simulink model "simulator"  (R2024a)
settings: Solver=VariableStepAuto  StartTime=0.0  StopTime=10  RelTol=1e-3
undefined symbols (not defined in the file): desiredState, gains, params, x0
libraries: simulink x2, matrix_library x1
settings Model: Creator=matteocolussi  LastModifiedBy=matteocolussi

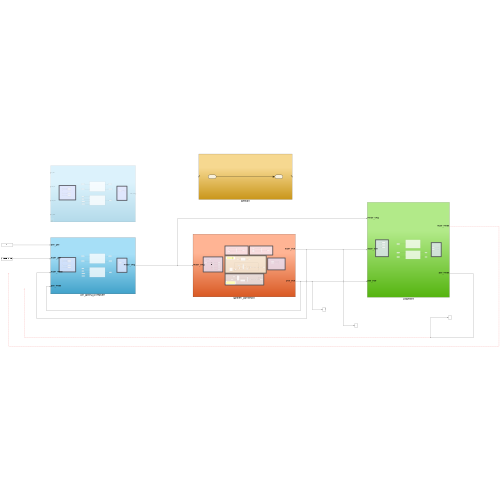
[thumbnail: Simulink's stored preview of the top-level diagram]
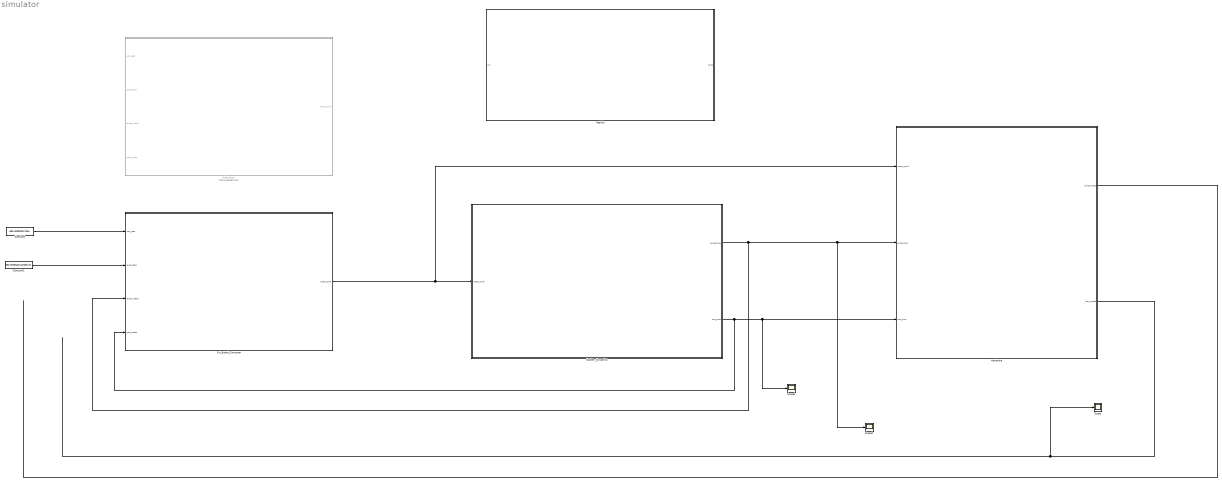
== system simulator ==
  Constant : Constant  Value=desiredState.rDes
  Constant1 : Constant  Value=desiredState.attDes(3)
  Hardware : Subsystem
  On_Board_Computer : Subsystem
  Results : Subsystem
  Scope : Scope
  Scope1 : Scope
  Scope2 : Scope
  Subsystem : Subsystem  Commented=on
  System_Dynamics : Subsystem
  wires:
  System_Dynamics/1(euler_true) -> On_Board_Computer/3(euler_meas), Hardware/2(euler_true), Scope2/1
  System_Dynamics/2(pos_true) -> On_Board_Computer/4(pos_meas), Hardware/3(pos_true), Scope1/1
  Hardware/1(euler_meas) -> ?
  Hardware/2(pos_meas) -> Scope/1
  Constant/1 -> On_Board_Computer/1(pos_des)
  Constant1/1 -> On_Board_Computer/2(euler_des)
  On_Board_Computer/1(motor_cmd) -> System_Dynamics/1(motor_cmd), Hardware/1(motor_cmd)

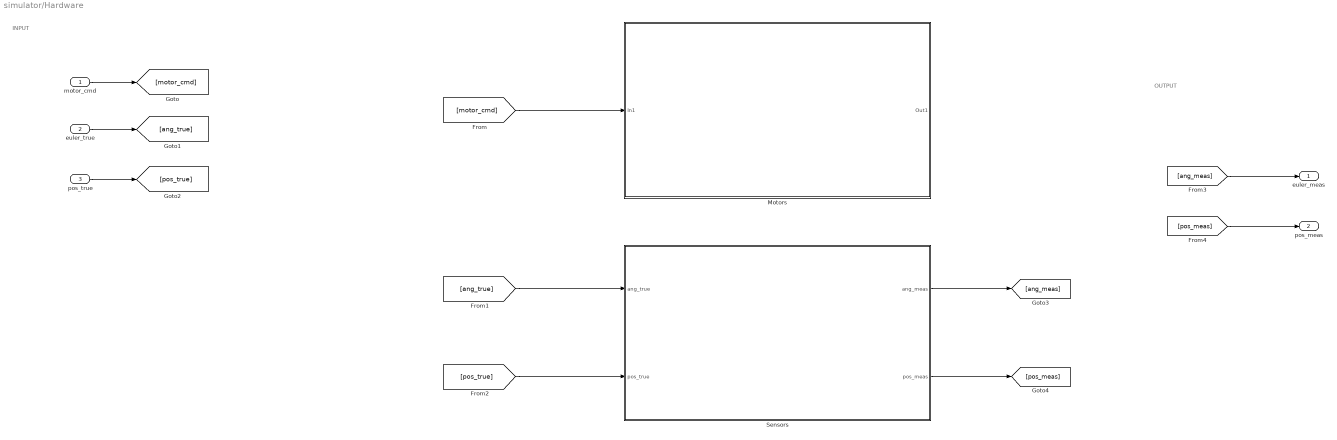
== system simulator/Hardware ==
  note: INPUT
  note: OUTPUT
  motor_cmd : Inport
  euler_true : Inport  Port=2
  pos_true : Inport  Port=3
  Motors : Subsystem
  Sensors : Subsystem
  euler_meas : Outport
  pos_meas : Outport  Port=2
  wires:
  motor_cmd/1 -> [motor_cmd]
  [motor_cmd] -> Motors/1(In1)
  euler_true/1 -> [ang_true]
  pos_true/1 -> [pos_true]
  [ang_true] -> Sensors/1(ang_true)
  [pos_true] -> Sensors/2(pos_true)
  Sensors/1(ang_meas) -> [ang_meas]
  Sensors/2(pos_meas) -> [pos_meas]
  [ang_meas] -> euler_meas/1
  [pos_meas] -> pos_meas/1

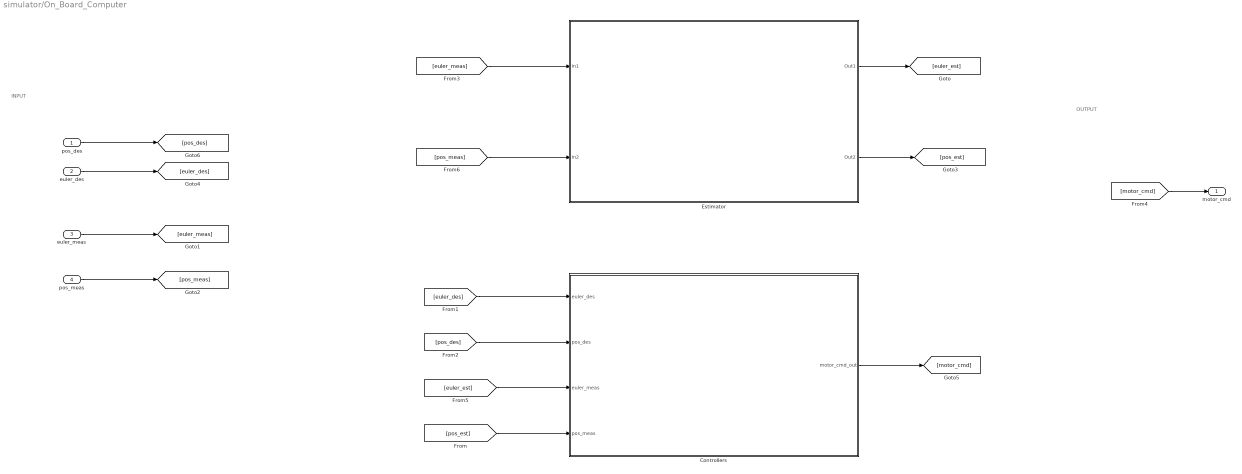
== system simulator/On_Board_Computer ==
  note: INPUT
  note: OUTPUT
  pos_des : Inport
  euler_des : Inport  Port=2
  euler_meas : Inport  Port=3
  pos_meas : Inport  Port=4
  Controllers : Subsystem
  Estimator : Subsystem
  motor_cmd : Outport
  wires:
  [euler_des] -> Controllers/1(euler_des)
  pos_des/1 -> [pos_des]
  pos_meas/1 -> [pos_meas]
  [pos_meas] -> Estimator/2(In2)
  [euler_meas] -> Estimator/1(In1)
  [pos_est] -> Controllers/4(pos_meas)
  euler_meas/1 -> [euler_meas]
  [motor_cmd] -> motor_cmd/1
  euler_des/1 -> [euler_des]
  [pos_des] -> Controllers/2(pos_des)
  Estimator/2(Out2) -> [pos_est]
  Estimator/1(Out1) -> [euler_est]
  [euler_est] -> Controllers/3(euler_meas)
  Controllers/1(motor_cmd_out) -> [motor_cmd]

== system simulator/Results ==
  In1 : Inport
  Out1 : Outport
  wires:
  In1/1 -> Out1/1

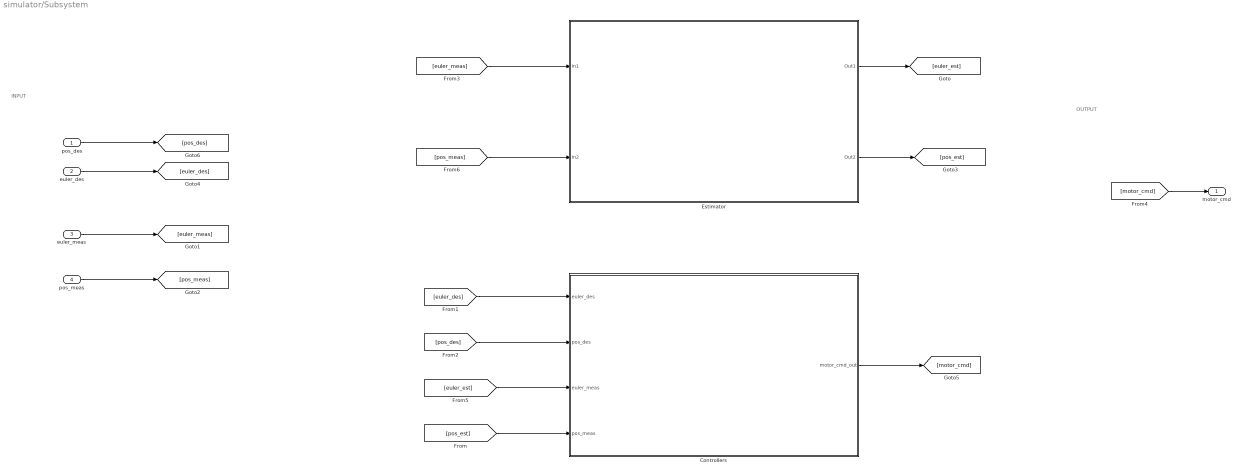
== system simulator/Subsystem ==
  note: INPUT
  note: OUTPUT
  pos_des : Inport
  euler_des : Inport  Port=2
  euler_meas : Inport  Port=3
  pos_meas : Inport  Port=4
  Controllers : Subsystem
  Estimator : Subsystem
  motor_cmd : Outport
  wires:
  [euler_des] -> Controllers/1(euler_des)
  pos_des/1 -> [pos_des]
  pos_meas/1 -> [pos_meas]
  [pos_meas] -> Estimator/2(In2)
  [euler_meas] -> Estimator/1(In1)
  [pos_est] -> Controllers/4(pos_meas)
  euler_meas/1 -> [euler_meas]
  [motor_cmd] -> motor_cmd/1
  euler_des/1 -> [euler_des]
  [pos_des] -> Controllers/2(pos_des)
  Estimator/2(Out2) -> [pos_est]
  Estimator/1(Out1) -> [euler_est]
  [euler_est] -> Controllers/3(euler_meas)
  Controllers/1(motor_cmd_out) -> [motor_cmd]

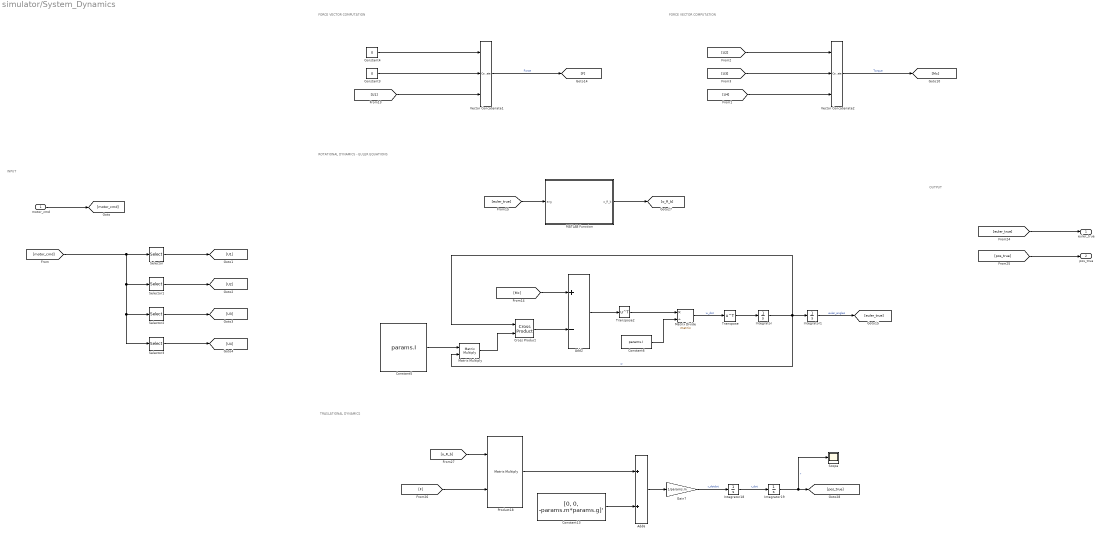
== system simulator/System_Dynamics ==
  note: ROTATIONAL DYNAMICS - EULER EQUATIONS
  note: FORCE VECTOR COMPUTATION
  note: INPUT
  note: OUTPUT
  note: TRASLATIONAL DYNAMICS
  note: FORCE VECTOR COMPUTATION
  motor_cmd : Inport
  Add2 : Sum  Inputs=+-
  Add6 : Sum
  Constant13 : Constant  Value=[0, 0, -params.m*params.g]'
  Constant3 : Constant  Value=0
  Constant4 : Constant  Value=0
  Constant5 : Constant  Value=params.I  VectorParams1D=off
  Constant6 : Constant  Value=params.I
  Cross Product : matrix_library/Cross Product
  Gain7 : Gain  Gain=1/params.m
  Integrator : Integrator
  Integrator1 : Integrator  InitialCondition=x0(7:9)
  Integrator18 : Integrator
  Integrator19 : Integrator  InitialCondition=x0(1:3);
  MATLAB Function : MATLAB Function  TreatAsAtomicUnit=on
  Matrix Divide : Product  Inputs=*/  Multiplication=Matrix(*)
  Matrix Multiply : Product  Multiplication=Matrix(*)
  Product18 : Product  Multiplication=Matrix(*)
  Scope : Scope
  Selector : Selector  InputPortWidth=4  IndexOptions=Index vector (dialog)  Indices=1  OutputSizes=1
  Selector1 : Selector  InputPortWidth=4  IndexOptions=Index vector (dialog)  Indices=2  OutputSizes=1
  Selector2 : Selector  InputPortWidth=4  IndexOptions=Index vector (dialog)  Indices=3  OutputSizes=1
  Selector3 : Selector  InputPortWidth=4  IndexOptions=Index vector (dialog)  Indices=4  OutputSizes=1
  Transpose : Math  Operator=transpose
  Transpose2 : Math  Operator=transpose
  Vector Concatenate1 : Concatenate  NumInputs=3
  Vector Concatenate2 : Concatenate  NumInputs=3
  euler_true : Outport
  pos_true : Outport  Port=2
  wires:
  motor_cmd/1 -> [motor_cmd]
  Selector/1 -> [U1]
  Selector1/1 -> [U2]
  Selector2/1 -> [U3]
  [motor_cmd] -> Selector3/1, Selector2/1, Selector1/1, Selector/1
  Selector3/1 -> [U4]
  [U1] -> Vector Concatenate1/3
  Constant3/1 -> Vector Concatenate1/2
  Constant4/1 -> Vector Concatenate1/1
  Vector Concatenate1/1 -> [F]  "Force"
  [euler_true] -> MATLAB Function/1(ang)
  MATLAB Function/1(o_R_b) -> [o_R_b]
  [euler_true] -> euler_true/1
  [pos_true] -> pos_true/1
  Add6/1 -> Gain7/1
  [F] -> Product18/2
  Product18/1 -> Add6/1
  Gain7/1 -> Integrator18/1  "r_dotdot"
  [o_R_b] -> Product18/1
  Constant13/1 -> Add6/2
  Integrator18/1 -> Integrator19/1  "r_dot"
  Integrator19/1 -> [pos_true], Scope/1  "r"
  Constant5/1 -> Matrix Multiply/1
  Matrix Multiply/1 -> Cross Product/2
  Cross Product/1 -> Add2/2
  Add2/1 -> Transpose2/1
  Constant6/1 -> Matrix Divide/2
  Matrix Divide/1 -> Transpose/1  "w_dot"
  Integrator/1 -> Integrator1/1, Cross Product/1, Matrix Multiply/2  "w"
  Integrator1/1 -> [euler_true]  "euler_angles"
  [U2] -> Vector Concatenate2/1
  Vector Concatenate2/1 -> [Mc]  "Torque"
  [U4] -> Vector Concatenate2/3
  [U3] -> Vector Concatenate2/2
  Transpose/1 -> Integrator/1
  [Mc] -> Add2/1
  Transpose2/1 -> Matrix Divide/1

== system simulator/Hardware/Motors ==
  In1 : Inport
  Out1 : Outport
  wires:
  In1/1 -> Out1/1

== system simulator/Hardware/Sensors ==
  note: OUTPUT
  note: INPUT
  ang_true : Inport
  pos_true : Inport  Port=2
  MPU6050 : Subsystem
  ang_meas : Outport
  pos_meas : Outport  Port=2
  wires:
  ang_true/1 -> [ang_true]
  pos_true/1 -> [pos_true]
  [ang_meas] -> ang_meas/1
  [pos_meas] -> pos_meas/1
  [ang_true] -> MPU6050/1(ang_true)
  [pos_true] -> MPU6050/2(pos_true)
  MPU6050/1(ang_meas) -> [ang_meas]
  MPU6050/2(pos_meas) -> [pos_meas]

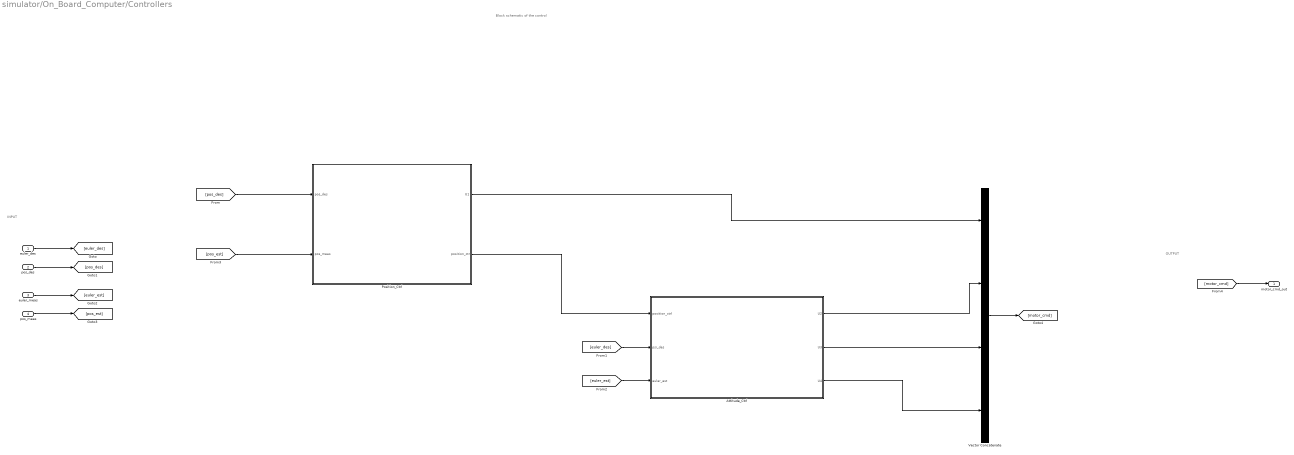
== system simulator/On_Board_Computer/Controllers ==
  note: Block schematic of the control
  note: OUTPUT
  note: INPUT
  euler_des : Inport
  pos_des : Inport  Port=2
  euler_meas : Inport  Port=3
  pos_meas : Inport  Port=4
  Attitude_Ctrl : Subsystem
  Position_Ctrl : Subsystem
  Vector Concatenate : Concatenate  NumInputs=4
  motor_cmd_out : Outport
  wires:
  euler_des/1 -> [euler_des]
  pos_des/1 -> [pos_des]
  pos_meas/1 -> [pos_est]
  euler_meas/1 -> [euler_est]
  [euler_est] -> Attitude_Ctrl/3(euler_est)
  [motor_cmd] -> motor_cmd_out/1
  [pos_est] -> Position_Ctrl/2(pos_meas)
  [pos_des] -> Position_Ctrl/1(pos_des)
  Position_Ctrl/2(position_ctrl) -> Attitude_Ctrl/1(position_ctrl)
  Position_Ctrl/1(U1) -> Vector Concatenate/1
  Attitude_Ctrl/1(U2) -> Vector Concatenate/2
  Attitude_Ctrl/2(U3) -> Vector Concatenate/3
  Attitude_Ctrl/3(U4) -> Vector Concatenate/4
  Vector Concatenate/1 -> [motor_cmd]
  [euler_des] -> Attitude_Ctrl/2(psi_des)

== system simulator/On_Board_Computer/Estimator ==
  In1 : Inport
  In2 : Inport  Port=2
  Out1 : Outport
  Out2 : Outport  Port=2
  wires:
  In1/1 -> Out1/1
  In2/1 -> Out2/1

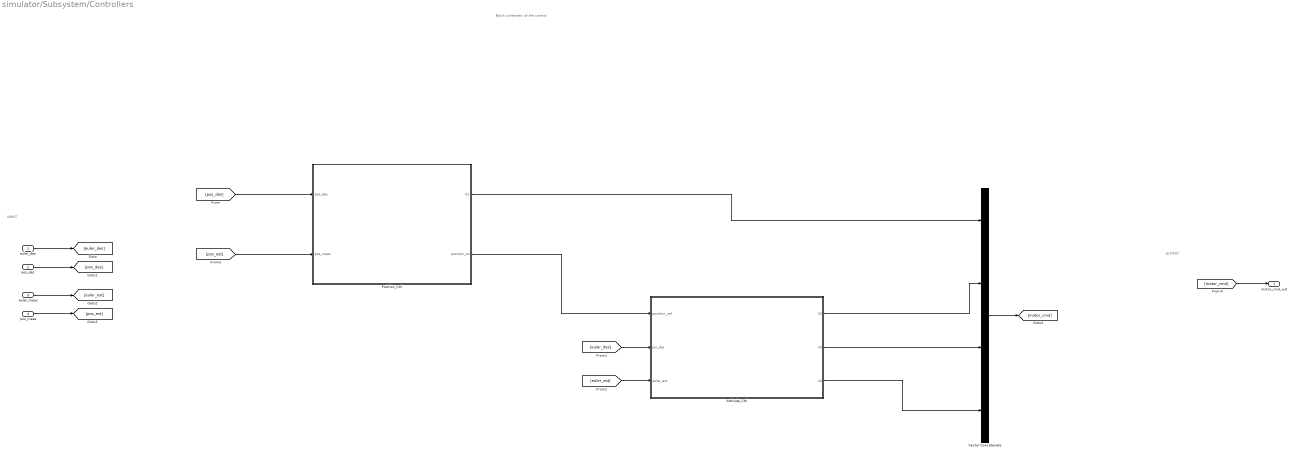
== system simulator/Subsystem/Controllers ==
  note: Block schematic of the control
  note: OUTPUT
  note: INPUT
  euler_des : Inport
  pos_des : Inport  Port=2
  euler_meas : Inport  Port=3
  pos_meas : Inport  Port=4
  Attitude_Ctrl : Subsystem
  Position_Ctrl : Subsystem
  Vector Concatenate : Concatenate  NumInputs=4
  motor_cmd_out : Outport
  wires:
  euler_des/1 -> [euler_des]
  pos_des/1 -> [pos_des]
  pos_meas/1 -> [pos_est]
  euler_meas/1 -> [euler_est]
  [euler_est] -> Attitude_Ctrl/3(euler_est)
  [motor_cmd] -> motor_cmd_out/1
  [pos_est] -> Position_Ctrl/2(pos_meas)
  [pos_des] -> Position_Ctrl/1(pos_des)
  Position_Ctrl/2(position_ctrl) -> Attitude_Ctrl/1(position_ctrl)
  Position_Ctrl/1(U1) -> Vector Concatenate/1
  Attitude_Ctrl/1(U2) -> Vector Concatenate/2
  Attitude_Ctrl/2(U3) -> Vector Concatenate/3
  Attitude_Ctrl/3(U4) -> Vector Concatenate/4
  Vector Concatenate/1 -> [motor_cmd]
  [euler_des] -> Attitude_Ctrl/2(psi_des)

== system simulator/Subsystem/Estimator ==
  In1 : Inport
  In2 : Inport  Port=2
  Out1 : Outport
  Out2 : Outport  Port=2
  wires:
  In1/1 -> Out1/1
  In2/1 -> Out2/1

== system simulator/Hardware/Sensors/MPU6050 ==
  note: INPUT
  note: OUTPUT
  ang_true : Inport
  pos_true : Inport  Port=2
  ACCELEROMETER : Subsystem
  GYROSCOPE : Subsystem
  ang_meas : Outport
  pos_meas : Outport  Port=2
  wires:
  ang_true/1 -> [ang_true]
  pos_true/1 -> [pos_true]
  [pos_meas] -> pos_meas/1
  [ang_meas] -> ang_meas/1
  [ang_true] -> GYROSCOPE/1(ang_true)
  [pos_true] -> ACCELEROMETER/1(pos_true)
  GYROSCOPE/1(ang_meas) -> [ang_meas]
  ACCELEROMETER/1(pos_meas) -> [pos_meas]

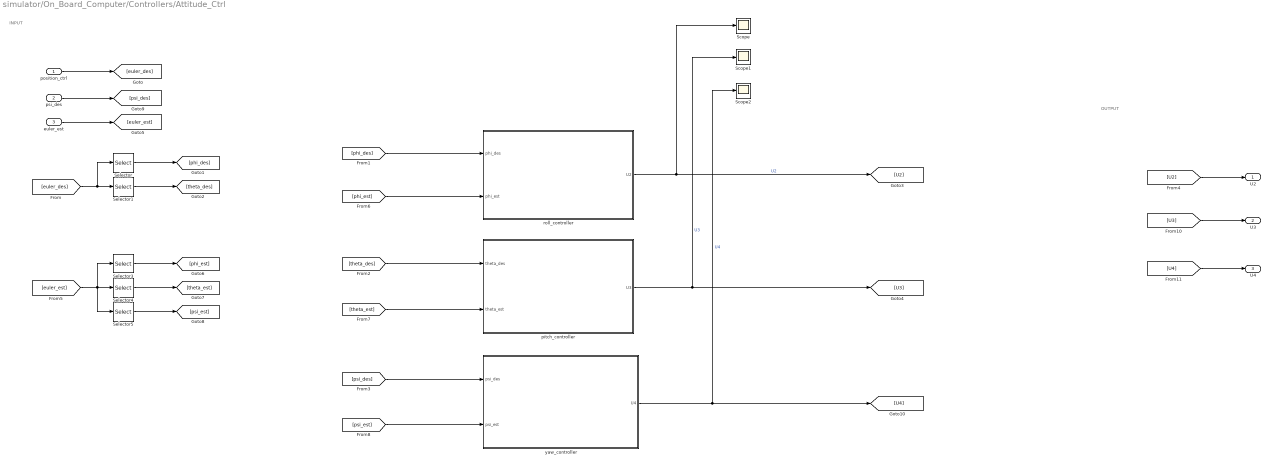
== system simulator/On_Board_Computer/Controllers/Attitude_Ctrl ==
  note: OUTPUT
  note: INPUT
  position_ctrl : Inport
  psi_des : Inport  Port=2
  euler_est : Inport  Port=3
  Scope : Scope
  Scope1 : Scope
  Scope2 : Scope
  Selector : Selector  InputPortWidth=2  IndexOptions=Index vector (dialog)  Indices=1  OutputSizes=1
  Selector1 : Selector  InputPortWidth=2  IndexOptions=Index vector (dialog)  Indices=2  OutputSizes=1
  Selector3 : Selector  InputPortWidth=3  IndexOptions=Index vector (dialog)  Indices=1  OutputSizes=1
  Selector4 : Selector  InputPortWidth=3  IndexOptions=Index vector (dialog)  Indices=2  OutputSizes=1
  Selector5 : Selector  InputPortWidth=3  IndexOptions=Index vector (dialog)  Indices=3  OutputSizes=1
  pitch_controller : Subsystem
  roll_controller : Subsystem
  yaw_controller : Subsystem
  U2 : Outport
  U3 : Outport  Port=2
  U4 : Outport  Port=3
  wires:
  position_ctrl/1 -> [euler_des]
  [phi_des] -> roll_controller/1(phi_des)
  [theta_des] -> pitch_controller/1(theta_des)
  [psi_des] -> yaw_controller/1(psi_des)
  roll_controller/1(U2) -> [U2], Scope/1  "U2"
  pitch_controller/1(U3) -> [U3], Scope1/1  "U3"
  yaw_controller/1(U4) -> [U4], Scope2/1  "U4"
  euler_est/1 -> [euler_est]
  [phi_est] -> roll_controller/2(phi_est)
  [theta_est] -> pitch_controller/2(theta_est)
  [psi_est] -> yaw_controller/2(psi_est)
  Selector/1 -> [phi_des]
  [euler_des] -> Selector1/1, Selector/1
  Selector1/1 -> [theta_des]
  [euler_est] -> Selector5/1, Selector4/1, Selector3/1
  Selector4/1 -> [theta_est]
  Selector5/1 -> [psi_est]
  Selector3/1 -> [phi_est]
  [U2] -> U2/1
  [U3] -> U3/1
  [U4] -> U4/1
  psi_des/1 -> [psi_des]

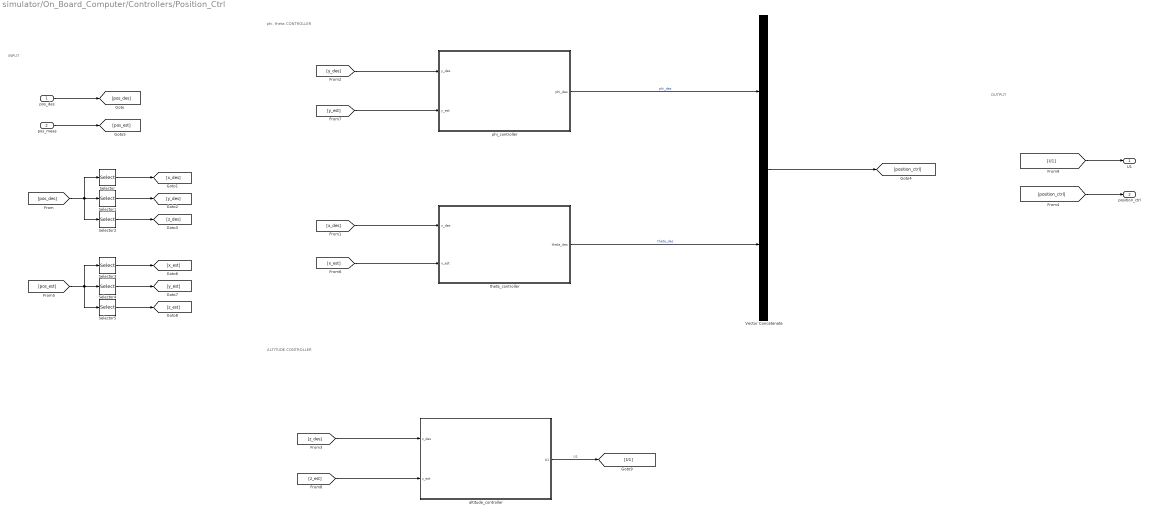
== system simulator/On_Board_Computer/Controllers/Position_Ctrl ==
  note: ALTITUDE CONTROLLER
  note: phi, theta CONTROLLER
  note: INPUT
  note: OUTPUT
  pos_des : Inport
  pos_meas : Inport  Port=2
  Selector : Selector  InputPortWidth=3  IndexOptions=Index vector (dialog)  Indices=1  OutputSizes=1
  Selector1 : Selector  InputPortWidth=3  IndexOptions=Index vector (dialog)  Indices=2  OutputSizes=1
  Selector2 : Selector  InputPortWidth=3  IndexOptions=Index vector (dialog)  Indices=3  OutputSizes=1
  Selector3 : Selector  InputPortWidth=3  IndexOptions=Index vector (dialog)  Indices=1  OutputSizes=1
  Selector4 : Selector  InputPortWidth=3  IndexOptions=Index vector (dialog)  Indices=2  OutputSizes=1
  Selector5 : Selector  InputPortWidth=3  IndexOptions=Index vector (dialog)  Indices=3  OutputSizes=1
  Vector Concatenate : Concatenate
  altitude_controller : Subsystem
  phi_controller : Subsystem
  theta_controller : Subsystem
  U1 : Outport
  position_ctrl : Outport  Port=2
  wires:
  Selector3/1 -> [x_est]
  Selector4/1 -> [y_est]
  [pos_est] -> Selector5/1, Selector4/1, Selector3/1
  pos_meas/1 -> [pos_est]
  Selector5/1 -> [z_est]
  [pos_des] -> Selector2/1, Selector1/1, Selector/1
  Selector/1 -> [x_des]
  pos_des/1 -> [pos_des]
  Selector1/1 -> [y_des]
  Selector2/1 -> [z_des]
  [y_est] -> phi_controller/2(y_est)
  [x_des] -> theta_controller/1(x_des)
  [y_des] -> phi_controller/1(y_des)
  [x_est] -> theta_controller/2(x_est)
  [position_ctrl] -> position_ctrl/1
  Vector Concatenate/1 -> [position_ctrl]
  theta_controller/1(theta_des) -> Vector Concatenate/2  "theta_des"
  [z_est] -> altitude_controller/2(z_est)
  [z_des] -> altitude_controller/1(z_des)
  altitude_controller/1(U1) -> [U1]  "U1"
  [U1] -> U1/1
  phi_controller/1(phi_des) -> Vector Concatenate/1  "phi_des"

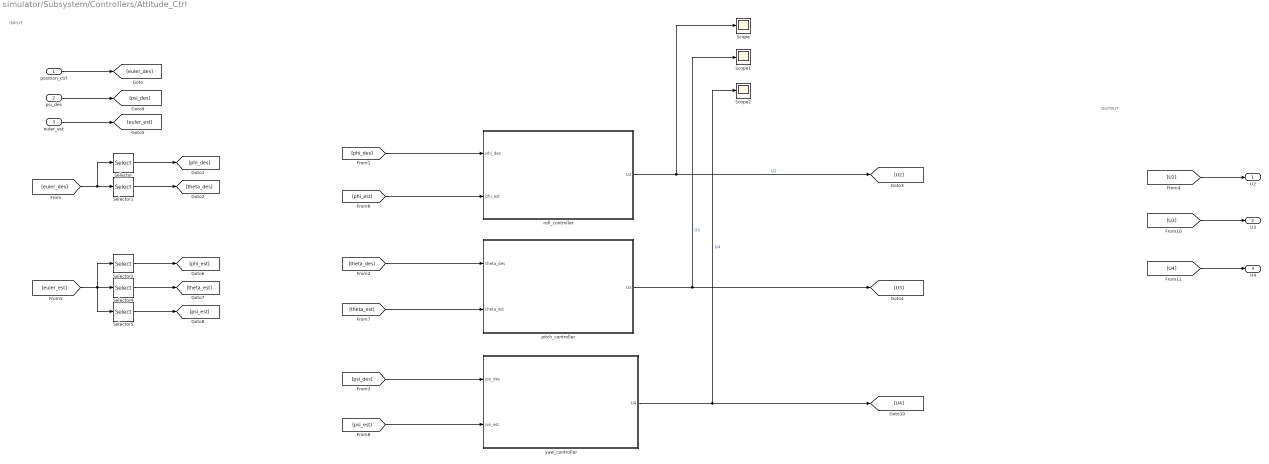
== system simulator/Subsystem/Controllers/Attitude_Ctrl ==
  note: OUTPUT
  note: INPUT
  position_ctrl : Inport
  psi_des : Inport  Port=2
  euler_est : Inport  Port=3
  Scope : Scope
  Scope1 : Scope
  Scope2 : Scope
  Selector : Selector  InputPortWidth=2  IndexOptions=Index vector (dialog)  Indices=1  OutputSizes=1
  Selector1 : Selector  InputPortWidth=2  IndexOptions=Index vector (dialog)  Indices=2  OutputSizes=1
  Selector3 : Selector  InputPortWidth=3  IndexOptions=Index vector (dialog)  Indices=1  OutputSizes=1
  Selector4 : Selector  InputPortWidth=3  IndexOptions=Index vector (dialog)  Indices=2  OutputSizes=1
  Selector5 : Selector  InputPortWidth=3  IndexOptions=Index vector (dialog)  Indices=3  OutputSizes=1
  pitch_controller : Subsystem
  roll_controller : Subsystem
  yaw_controller : Subsystem
  U2 : Outport
  U3 : Outport  Port=2
  U4 : Outport  Port=3
  wires:
  position_ctrl/1 -> [euler_des]
  [phi_des] -> roll_controller/1(phi_des)
  [theta_des] -> pitch_controller/1(theta_des)
  [psi_des] -> yaw_controller/1(psi_des)
  roll_controller/1(U2) -> [U2], Scope/1  "U2"
  pitch_controller/1(U3) -> [U3], Scope1/1  "U3"
  yaw_controller/1(U4) -> [U4], Scope2/1  "U4"
  euler_est/1 -> [euler_est]
  [phi_est] -> roll_controller/2(phi_est)
  [theta_est] -> pitch_controller/2(theta_est)
  [psi_est] -> yaw_controller/2(psi_est)
  Selector/1 -> [phi_des]
  [euler_des] -> Selector1/1, Selector/1
  Selector1/1 -> [theta_des]
  [euler_est] -> Selector5/1, Selector4/1, Selector3/1
  Selector4/1 -> [theta_est]
  Selector5/1 -> [psi_est]
  Selector3/1 -> [phi_est]
  [U2] -> U2/1
  [U3] -> U3/1
  [U4] -> U4/1
  psi_des/1 -> [psi_des]

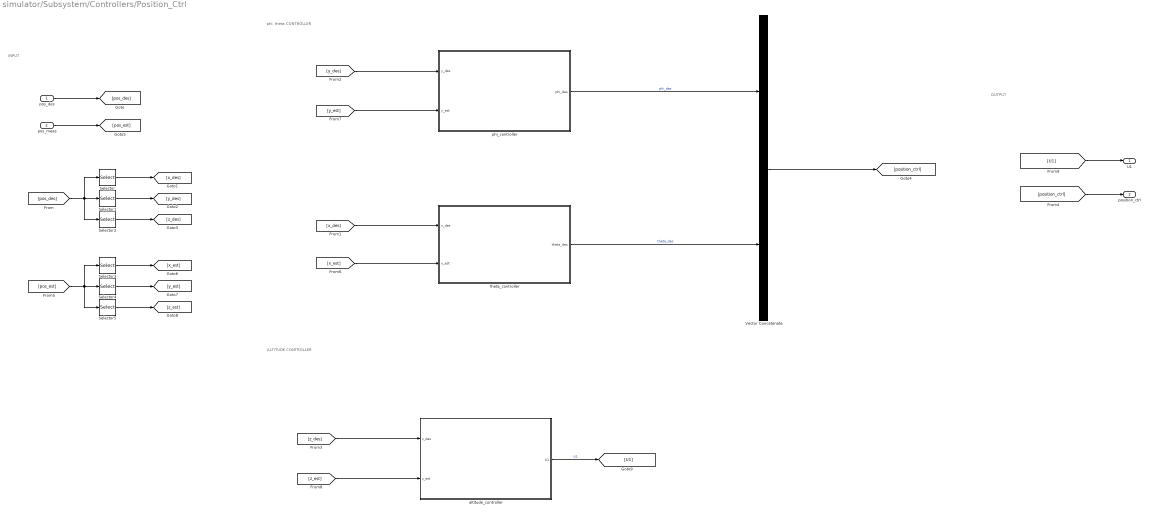
== system simulator/Subsystem/Controllers/Position_Ctrl ==
  note: ALTITUDE CONTROLLER
  note: phi, theta CONTROLLER
  note: INPUT
  note: OUTPUT
  pos_des : Inport
  pos_meas : Inport  Port=2
  Selector : Selector  InputPortWidth=3  IndexOptions=Index vector (dialog)  Indices=1  OutputSizes=1
  Selector1 : Selector  InputPortWidth=3  IndexOptions=Index vector (dialog)  Indices=2  OutputSizes=1
  Selector2 : Selector  InputPortWidth=3  IndexOptions=Index vector (dialog)  Indices=3  OutputSizes=1
  Selector3 : Selector  InputPortWidth=3  IndexOptions=Index vector (dialog)  Indices=1  OutputSizes=1
  Selector4 : Selector  InputPortWidth=3  IndexOptions=Index vector (dialog)  Indices=2  OutputSizes=1
  Selector5 : Selector  InputPortWidth=3  IndexOptions=Index vector (dialog)  Indices=3  OutputSizes=1
  Vector Concatenate : Concatenate
  altitude_controller : Subsystem
  phi_controller : Subsystem
  theta_controller : Subsystem
  U1 : Outport
  position_ctrl : Outport  Port=2
  wires:
  Selector3/1 -> [x_est]
  Selector4/1 -> [y_est]
  [pos_est] -> Selector5/1, Selector4/1, Selector3/1
  pos_meas/1 -> [pos_est]
  Selector5/1 -> [z_est]
  [pos_des] -> Selector2/1, Selector1/1, Selector/1
  Selector/1 -> [x_des]
  pos_des/1 -> [pos_des]
  Selector1/1 -> [y_des]
  Selector2/1 -> [z_des]
  [y_est] -> phi_controller/2(y_est)
  [x_des] -> theta_controller/1(x_des)
  [y_des] -> phi_controller/1(y_des)
  [x_est] -> theta_controller/2(x_est)
  [position_ctrl] -> position_ctrl/1
  Vector Concatenate/1 -> [position_ctrl]
  theta_controller/1(theta_des) -> Vector Concatenate/2  "theta_des"
  [z_est] -> altitude_controller/2(z_est)
  [z_des] -> altitude_controller/1(z_des)
  altitude_controller/1(U1) -> [U1]  "U1"
  [U1] -> U1/1
  phi_controller/1(phi_des) -> Vector Concatenate/1  "phi_des"

== system simulator/Hardware/Sensors/MPU6050/ACCELEROMETER ==
  pos_true : Inport
  Band-Limited White Noise : simulink/Sources/Band-Limited White Noise  Cov=[0.1]  Ts=0.1  seed=[23341]
  Sum : Sum  Inputs=|++
  pos_meas : Outport
  wires:
  Band-Limited White Noise/1 -> Sum/2
  pos_true/1 -> Sum/1
  Sum/1 -> pos_meas/1

== system simulator/Hardware/Sensors/MPU6050/GYROSCOPE ==
  ang_true : Inport
  Band-Limited White Noise : simulink/Sources/Band-Limited White Noise  Cov=[0.1]  Ts=0.1  seed=[23341]
  Sum : Sum  Inputs=|++
  ang_meas : Outport
  wires:
  ang_true/1 -> Sum/1
  Band-Limited White Noise/1 -> Sum/2
  Sum/1 -> ang_meas/1

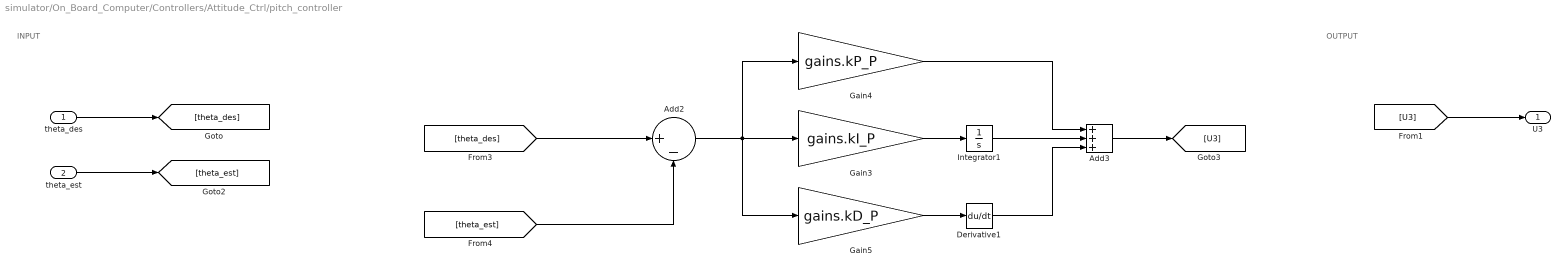
== system simulator/On_Board_Computer/Controllers/Attitude_Ctrl/pitch_controller ==
  note: OUTPUT
  note: INPUT
  theta_des : Inport
  theta_est : Inport  Port=2
  Add2 : Sum  Inputs=|+-
  Add3 : Sum  Inputs=+++
  Derivative1 : Derivative
  Gain3 : Gain  Gain=gains.kI_P
  Gain4 : Gain  Gain=gains.kP_P
  Gain5 : Gain  Gain=gains.kD_P
  Integrator1 : Integrator
  U3 : Outport
  wires:
  [U3] -> U3/1
  theta_des/1 -> [theta_des]
  theta_est/1 -> [theta_est]
  [theta_des] -> Add2/1
  Gain4/1 -> Add3/1
  Add3/1 -> [U3]
  Derivative1/1 -> Add3/3
  [theta_est] -> Add2/2
  Integrator1/1 -> Add3/2
  Add2/1 -> Gain5/1, Gain4/1, Gain3/1
  Gain5/1 -> Derivative1/1
  Gain3/1 -> Integrator1/1

== system simulator/On_Board_Computer/Controllers/Attitude_Ctrl/roll_controller ==
  note: OUTPUT
  note: INPUT
  phi_des : Inport
  phi_est : Inport  Port=2
  Add2 : Sum  Inputs=|+-
  Add3 : Sum  Inputs=+++
  Derivative1 : Derivative
  Gain3 : Gain  Gain=gains.kI_R
  Gain4 : Gain  Gain=gains.kP_R
  Gain5 : Gain  Gain=gains.kD_R
  Integrator1 : Integrator
  U2 : Outport
  wires:
  phi_des/1 -> [phi_des]
  [U2] -> U2/1
  phi_est/1 -> [phi_est]
  [phi_des] -> Add2/1
  Gain4/1 -> Add3/1
  Add3/1 -> [U2]
  Derivative1/1 -> Add3/3
  [phi_est] -> Add2/2
  Integrator1/1 -> Add3/2
  Add2/1 -> Gain5/1, Gain4/1, Gain3/1
  Gain5/1 -> Derivative1/1
  Gain3/1 -> Integrator1/1

== system simulator/On_Board_Computer/Controllers/Attitude_Ctrl/yaw_controller ==
  note: OUTPUT
  note: INPUT
  psi_des : Inport
  psi_est : Inport  Port=2
  Add2 : Sum  Inputs=|+-
  Add3 : Sum  Inputs=+++
  Derivative1 : Derivative
  Gain3 : Gain  Gain=gains.kI_Y
  Gain4 : Gain  Gain=gains.kP_Y
  Gain5 : Gain  Gain=gains.kD_Y
  Integrator1 : Integrator
  U4 : Outport
  wires:
  [U4] -> U4/1
  psi_des/1 -> [psi_des]
  psi_est/1 -> [psi_est]
  [psi_des] -> Add2/1
  Gain4/1 -> Add3/1
  Add3/1 -> [U4]
  Derivative1/1 -> Add3/3
  [psi_est] -> Add2/2
  Integrator1/1 -> Add3/2
  Add2/1 -> Gain5/1, Gain4/1, Gain3/1
  Gain5/1 -> Derivative1/1
  Gain3/1 -> Integrator1/1

== system simulator/On_Board_Computer/Controllers/Position_Ctrl/altitude_controller ==
  note: OUTPUT
  note: INPUT
  z_des : Inport
  z_est : Inport  Port=2
  Add2 : Sum  Inputs=|+-
  Add3 : Sum  Inputs=+++
  Derivative1 : Derivative
  Gain3 : Gain  Gain=gains.kI_T
  Gain4 : Gain  Gain=gains.kP_T
  Gain5 : Gain  Gain=gains.kD_T
  Integrator1 : Integrator
  U1 : Outport
  wires:
  [U1] -> U1/1
  z_des/1 -> [z_des]
  z_est/1 -> [z_est]
  [z_des] -> Add2/1
  Gain4/1 -> Add3/1
  Add3/1 -> [U1]
  Derivative1/1 -> Add3/3
  [z_est] -> Add2/2
  Integrator1/1 -> Add3/2
  Add2/1 -> Gain5/1, Gain4/1, Gain3/1
  Gain5/1 -> Derivative1/1
  Gain3/1 -> Integrator1/1

== system simulator/On_Board_Computer/Controllers/Position_Ctrl/phi_controller ==
  note: OUTPUT
  note: INPUT
  y_des : Inport
  y_est : Inport  Port=2
  Add : Sum  Inputs=|+-
  Add1 : Sum  Inputs=+++
  Derivative : Derivative
  Gain1 : Gain  Gain=gains.kI_phi
  Gain2 : Gain  Gain=gains.kP_phi
  Gain3 : Gain  Gain=gains.kD_phi
  Integrator : Integrator
  phi_des : Outport
  wires:
  [phi_des] -> phi_des/1
  [y_des] -> Add/1
  y_des/1 -> [y_des]
  y_est/1 -> [y_est]
  [y_est] -> Add/2
  Integrator/1 -> Add1/2
  Gain1/1 -> Integrator/1
  Add/1 -> Gain3/1, Gain2/1, Gain1/1
  Gain2/1 -> Add1/1
  Derivative/1 -> Add1/3
  Add1/1 -> [phi_des]
  Gain3/1 -> Derivative/1

== system simulator/On_Board_Computer/Controllers/Position_Ctrl/theta_controller ==
  note: OUTPUT
  note: INPUT
  x_des : Inport
  x_est : Inport  Port=2
  Add2 : Sum  Inputs=|+-
  Add3 : Sum  Inputs=+++
  Derivative1 : Derivative
  Gain3 : Gain  Gain=gains.kI_theta
  Gain4 : Gain  Gain=gains.kP_theta
  Gain5 : Gain  Gain=gains.kD_theta
  Integrator1 : Integrator
  theta_des : Outport
  wires:
  x_des/1 -> [x_des]
  [theta_des] -> theta_des/1
  x_est/1 -> [x_est]
  [x_des] -> Add2/1
  Gain4/1 -> Add3/1
  Add3/1 -> [theta_des]
  Derivative1/1 -> Add3/3
  [x_est] -> Add2/2
  Integrator1/1 -> Add3/2
  Add2/1 -> Gain5/1, Gain4/1, Gain3/1
  Gain5/1 -> Derivative1/1
  Gain3/1 -> Integrator1/1

== system simulator/Subsystem/Controllers/Attitude_Ctrl/pitch_controller ==
  note: OUTPUT
  note: INPUT
  theta_des : Inport
  theta_est : Inport  Port=2
  Add2 : Sum  Inputs=|+-
  Add3 : Sum  Inputs=+++
  Derivative1 : Derivative
  Gain3 : Gain  Gain=gains.kI_P
  Gain4 : Gain  Gain=gains.kP_P
  Gain5 : Gain  Gain=gains.kD_P
  Integrator1 : Integrator
  U3 : Outport
  wires:
  [U3] -> U3/1
  theta_des/1 -> [theta_des]
  theta_est/1 -> [theta_est]
  [theta_des] -> Add2/1
  Gain4/1 -> Add3/1
  Add3/1 -> [U3]
  Derivative1/1 -> Add3/3
  [theta_est] -> Add2/2
  Integrator1/1 -> Add3/2
  Add2/1 -> Gain5/1, Gain4/1, Gain3/1
  Gain5/1 -> Derivative1/1
  Gain3/1 -> Integrator1/1

== system simulator/Subsystem/Controllers/Attitude_Ctrl/roll_controller ==
  note: OUTPUT
  note: INPUT
  phi_des : Inport
  phi_est : Inport  Port=2
  Add2 : Sum  Inputs=|+-
  Add3 : Sum  Inputs=+++
  Derivative1 : Derivative
  Gain3 : Gain  Gain=gains.kI_R
  Gain4 : Gain  Gain=gains.kP_R
  Gain5 : Gain  Gain=gains.kD_R
  Integrator1 : Integrator
  U2 : Outport
  wires:
  phi_des/1 -> [phi_des]
  [U2] -> U2/1
  phi_est/1 -> [phi_est]
  [phi_des] -> Add2/1
  Gain4/1 -> Add3/1
  Add3/1 -> [U2]
  Derivative1/1 -> Add3/3
  [phi_est] -> Add2/2
  Integrator1/1 -> Add3/2
  Add2/1 -> Gain5/1, Gain4/1, Gain3/1
  Gain5/1 -> Derivative1/1
  Gain3/1 -> Integrator1/1

== system simulator/Subsystem/Controllers/Attitude_Ctrl/yaw_controller ==
  note: OUTPUT
  note: INPUT
  psi_des : Inport
  psi_est : Inport  Port=2
  Add2 : Sum  Inputs=|+-
  Add3 : Sum  Inputs=+++
  Derivative1 : Derivative
  Gain3 : Gain  Gain=gains.kI_Y
  Gain4 : Gain  Gain=gains.kP_Y
  Gain5 : Gain  Gain=gains.kD_Y
  Integrator1 : Integrator
  U4 : Outport
  wires:
  [U4] -> U4/1
  psi_des/1 -> [psi_des]
  psi_est/1 -> [psi_est]
  [psi_des] -> Add2/1
  Gain4/1 -> Add3/1
  Add3/1 -> [U4]
  Derivative1/1 -> Add3/3
  [psi_est] -> Add2/2
  Integrator1/1 -> Add3/2
  Add2/1 -> Gain5/1, Gain4/1, Gain3/1
  Gain5/1 -> Derivative1/1
  Gain3/1 -> Integrator1/1

== system simulator/Subsystem/Controllers/Position_Ctrl/altitude_controller ==
  note: OUTPUT
  note: INPUT
  z_des : Inport
  z_est : Inport  Port=2
  Add2 : Sum  Inputs=|+-
  Add3 : Sum  Inputs=+++
  Derivative1 : Derivative
  Gain3 : Gain  Gain=gains.kI_T
  Gain4 : Gain  Gain=gains.kP_T
  Gain5 : Gain  Gain=gains.kD_T
  Integrator1 : Integrator
  U1 : Outport
  wires:
  [U1] -> U1/1
  z_des/1 -> [z_des]
  z_est/1 -> [z_est]
  [z_des] -> Add2/1
  Gain4/1 -> Add3/1
  Add3/1 -> [U1]
  Derivative1/1 -> Add3/3
  [z_est] -> Add2/2
  Integrator1/1 -> Add3/2
  Add2/1 -> Gain5/1, Gain4/1, Gain3/1
  Gain5/1 -> Derivative1/1
  Gain3/1 -> Integrator1/1

== system simulator/Subsystem/Controllers/Position_Ctrl/phi_controller ==
  note: OUTPUT
  note: INPUT
  y_des : Inport
  y_est : Inport  Port=2
  Add : Sum  Inputs=|+-
  Add1 : Sum  Inputs=+++
  Derivative : Derivative
  Gain1 : Gain  Gain=gains.kI_phi
  Gain2 : Gain  Gain=gains.kP_phi
  Gain3 : Gain  Gain=gains.kD_phi
  Integrator : Integrator
  phi_des : Outport
  wires:
  [phi_des] -> phi_des/1
  [y_des] -> Add/1
  y_des/1 -> [y_des]
  y_est/1 -> [y_est]
  [y_est] -> Add/2
  Integrator/1 -> Add1/2
  Gain1/1 -> Integrator/1
  Add/1 -> Gain3/1, Gain2/1, Gain1/1
  Gain2/1 -> Add1/1
  Derivative/1 -> Add1/3
  Add1/1 -> [phi_des]
  Gain3/1 -> Derivative/1

== system simulator/Subsystem/Controllers/Position_Ctrl/theta_controller ==
  note: OUTPUT
  note: INPUT
  x_des : Inport
  x_est : Inport  Port=2
  Add2 : Sum  Inputs=|+-
  Add3 : Sum  Inputs=+++
  Derivative1 : Derivative
  Gain3 : Gain  Gain=gains.kI_theta
  Gain4 : Gain  Gain=gains.kP_theta
  Gain5 : Gain  Gain=gains.kD_theta
  Integrator1 : Integrator
  theta_des : Outport
  wires:
  x_des/1 -> [x_des]
  [theta_des] -> theta_des/1
  x_est/1 -> [x_est]
  [x_des] -> Add2/1
  Gain4/1 -> Add3/1
  Add3/1 -> [theta_des]
  Derivative1/1 -> Add3/3
  [x_est] -> Add2/2
  Integrator1/1 -> Add3/2
  Add2/1 -> Gain5/1, Gain4/1, Gain3/1
  Gain5/1 -> Derivative1/1
  Gain3/1 -> Integrator1/1

== matlab function simulator/System_Dynamics/MATLAB Function ==
  data: ang input; o_R_b output
function o_R_b  = RotMatrix(ang)

phi = ang(1);
theta = ang(2);
psi = ang(3);

o_R_b = zeros(3,3);

R_psi = [cos(psi),          -sin(psi),          0;
         sin(psi),           cos(psi),          0;
                0,                  0,          1];

R_theta = [cos(theta),              0,          sin(theta);
                    0,              1,                   0;
          -sin(theta),              0,          cos(theta)];

R_phi = [1,             0,              0;
         0,      cos(phi),      -sin(phi);
         0,      sin(phi),       cos(phi)];

o_R_b = R_psi * R_theta * R_phi;

end
